simulink model "Copy_of_PROTOTIP_FULL2_plus_schema"  (R2022b)
settings: Solver=VariableStepAuto  StartTime=0.0  StopTime=5  FixedStep=1  RelTol=1e-3
model workspace (MAT data in the model file):
  K = Simulink.Parameter
  K.DataType = 'auto'
  K.Complexity = 'real'
  K.Dimensions = [0 0]
  K_v = Simulink.Parameter
  K_v.DataType = 'auto'
  K_v.Complexity = 'real'
  K_v.Dimensions = [0 0]
  Kp = Simulink.Parameter
  Kp.DataType = 'auto'
  Kp.Complexity = 'real'
  Kp.Dimensions = [0 0]
  Kv = Simulink.Parameter
  Kv.DataType = 'auto'
  Kv.Complexity = 'real'
  Kv.Dimensions = [0 0]
  Multiply1 = 1
  T2 = Simulink.Parameter
  T2.DataType = 'auto'
  T2.Complexity = 'real'
  T2.Dimensions = [0 0]
  W = Simulink.Parameter
  W.DataType = 'auto'
  W.Complexity = 'real'
  W.Dimensions = [0 0]
  q2dor = Simulink.Parameter
  q2dor.DataType = 'auto'
  q2dor.Complexity = 'real'
  q2dor.Dimensions = [0 0]
  q_1 = Simulink.Parameter
  q_1.Value = 1
  q_1.DataType = 'auto'
  q_1.Complexity = 'real'
  q_1.Dimensions = [1 1]
  q_1dor = Simulink.Parameter
  q_1dor.Value = 1
  q_1dor.DataType = 'auto'
  q_1dor.Complexity = 'real'
  q_1dor.Dimensions = [1 1]
  q_2dor = Simulink.Parameter
  q_2dor.Value = 1
  q_2dor.DataType = 'auto'
  q_2dor.Complexity = 'real'
  q_2dor.Dimensions = [1 1]
undefined symbols (not defined in the file or in its folder): X, Y, Z
libraries: sm_lib x17, nesl_utility x7
settings Model: Creator=Dell  LastModifiedBy=Dell
settings SimscapeCC: ExplicitSolverDiagnosticOptions=none

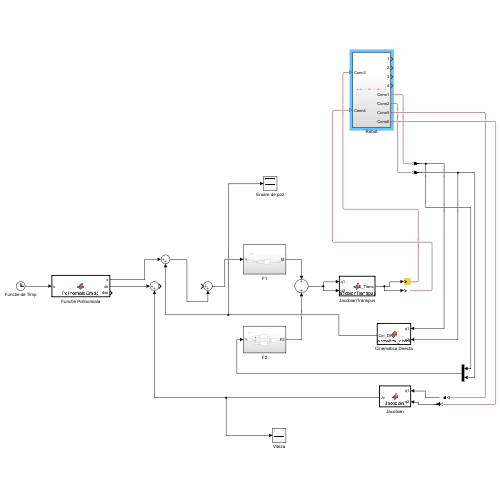
[thumbnail: Simulink's stored preview of the top-level diagram]
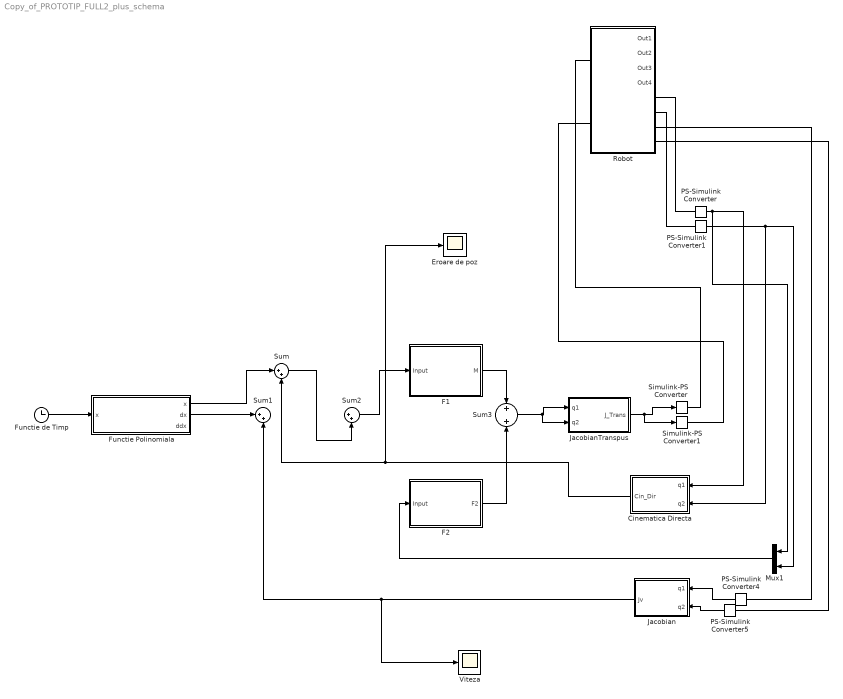
== system Copy_of_PROTOTIP_FULL2_plus_schema ==
  Cinematica Directa : MATLAB Function  TreatAsAtomicUnit=on
  Eroare de poz : Scope
  F1 : Subsystem
  F2 : Subsystem
  Functie Polinomiala : MATLAB Function  TreatAsAtomicUnit=on
  Functie de Timp : Clock
  Jacobian : MATLAB Function  TreatAsAtomicUnit=on
  JacobianTranspus : MATLAB Function  TreatAsAtomicUnit=on
  Mux1 : Mux  Inputs=2
  PS-Simulink Converter{,1,4..5} (4 alike) : nesl_utility/PS-Simulink Converter  PhysicalDomain=network_engine_domain  SubClassName=ps_output  LeftPortType=input  RightPortType=output  PseudoPeriodic=off  Frequencies=[]  VectorFormat=inherit  Unit=inherit  AffineConversion=off
  Robot : Subsystem
  Simulink-PS Converter : nesl_utility/Simulink-PS Converter  PhysicalDomain=network_engine_domain  SubClassName=ps_input  LeftPortType=input  RightPortType=output  PseudoPeriodic=off  Frequencies=[]  NoiseDistribution=none  NoiseParameters=[]  Unit=1  AffineConversion=on  FilteringAndDerivatives=provide  SimscapeFilterOrder=1  InputFilterTimeConstant=0.001  UdotUserProvided=0
  Simulink-PS Converter1 : nesl_utility/Simulink-PS Converter  PhysicalDomain=network_engine_domain  SubClassName=ps_input  LeftPortType=input  RightPortType=output  PseudoPeriodic=off  Frequencies=[]  NoiseDistribution=none  NoiseParameters=[]  Unit=1  AffineConversion=on  FilteringAndDerivatives=provide  SimscapeFilterOrder=1  InputFilterTimeConstant=0.001  UdotUserProvided=0
  Sum : Sum  Inputs=|++
  Sum1 : Sum  Inputs=|++
  Sum2 : Sum  Inputs=|++
  Sum3 : Sum  OutDataTypeStr=Inherit: Same as first input
  Viteza : Scope
  wires:
  Functie de Timp/1 -> Functie Polinomiala/1("x ")
  Functie Polinomiala/1(x) -> Sum/1
  F1/1(M) -> Sum3/1
  F2/1(F2) -> Sum3/2
  PS-Simulink Converter/1 -> Mux1/1, Cinematica Directa/1(q1)
  Cinematica Directa/1(Cin_Dir) -> Sum/2, Eroare de poz/1
  PS-Simulink Converter1/1 -> Mux1/2, Cinematica Directa/2(q2)
  Mux1/1 -> F2/1(Input)
  PS-Simulink Converter4/1 -> Jacobian/1(q1)
  PS-Simulink Converter5/1 -> Jacobian/2(q2)
  Functie Polinomiala/2(dx) -> Sum1/1
  Jacobian/1(Jv) -> Viteza/1, Sum1/2
  Sum2/1 -> F1/1(Input)
  JacobianTranspus/1(J_Trans) -> Simulink-PS Converter1/1, Simulink-PS Converter/1
  Sum/1 -> Sum2/2
  Sum3/1 -> JacobianTranspus/2(q2), JacobianTranspus/1(q1)
  connections:
  Simulink-PS Converter/RConn1 -- Robot/LConn1
  Simulink-PS Converter1/RConn1 -- Robot/LConn2
  PS-Simulink Converter/LConn1 -- Robot/RConn1
  Robot/RConn2 -- PS-Simulink Converter1/LConn1
  Robot/RConn3 -- PS-Simulink Converter4/LConn1
  Robot/RConn4 -- PS-Simulink Converter5/LConn1

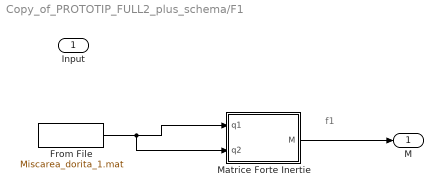
== system Copy_of_PROTOTIP_FULL2_plus_schema/F1 ==
  note: f1
  Input : Inport
  From File : FromFile  FileName=Miscarea_dorita_1.mat
  Matrice Forte Inertie : MATLAB Function  TreatAsAtomicUnit=on
  M : Outport
  wires:
  Matrice Forte Inertie/1(M) -> M/1
  From File/1 -> Matrice Forte Inertie/2(q2), Matrice Forte Inertie/1(q1)

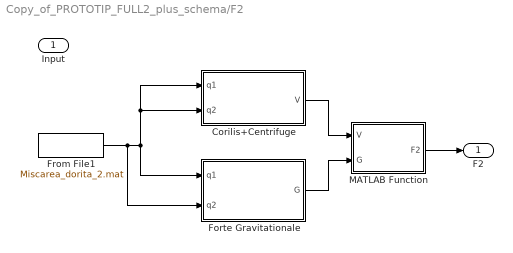
== system Copy_of_PROTOTIP_FULL2_plus_schema/F2 ==
  Input : Inport
  Corilis+Centrifuge : MATLAB Function  TreatAsAtomicUnit=on
  Forte Gravitationale : MATLAB Function  TreatAsAtomicUnit=on
  From File1 : FromFile  FileName=Miscarea_dorita_2.mat  SampleTime=0
  MATLAB Function : MATLAB Function  TreatAsAtomicUnit=on
  F2 : Outport
  wires:
  From File1/1 -> Forte Gravitationale/2(q2), Forte Gravitationale/1(q1), Corilis+Centrifuge/2(q2), Corilis+Centrifuge/1(q1)
  Corilis+Centrifuge/1(V) -> MATLAB Function/1(V)
  Forte Gravitationale/1(G) -> MATLAB Function/2(G)
  MATLAB Function/1(F2) -> F2/1

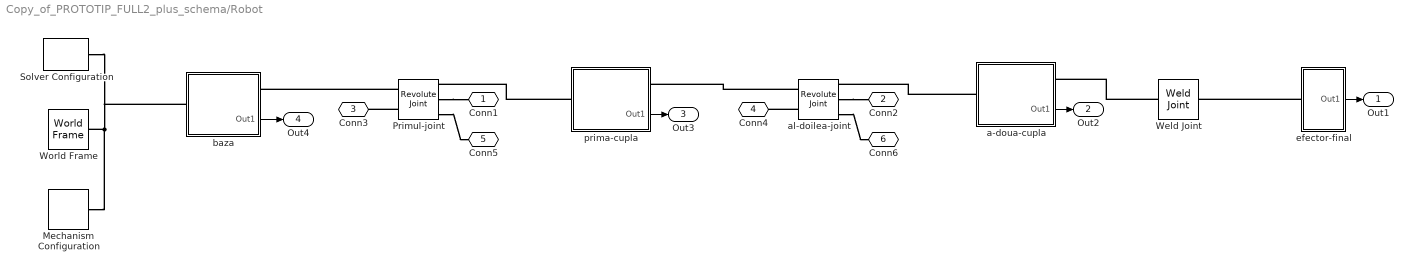
== system Copy_of_PROTOTIP_FULL2_plus_schema/Robot ==
  Mechanism Configuration : sm_lib/Utilities/Mechanism Configuration  UniformGravity=Constant  GravityVector=[0 0 -9.80665]  GravityUnits=m/s^2  LinearizationDelta=0.001  JointModeTransitionNonlinearIterations=2
  Primul-joint : sm_lib/Joints/Revolute Joint  JointMode=Normal  SenseConstraintForce=off  SenseConstraintForceX=off  SenseConstraintForceY=off  SenseConstraintForceZ=off  SenseConstraintTorque=off  SenseConstraintTorqueX=off  SenseConstraintTorqueY=off  SenseConstraintTorqueZ=off  SenseTotalForce=off  SenseTotalForceX=off  SenseTotalForceY=off  SenseTotalForceZ=off  SenseTotalTorque=off  SenseTotalTorqueX=off  SenseTotalTorqueY=off  SenseTotalTorqueZ=off  CompositeWrenchDir=FollowerOnBase  CompositeWrenchFrame=BaseFrame  EquilibriumPosition=0  EquilibriumPositionUnits=deg  SpringStiffness=0  SpringStiffnessUnits=N*m/deg  DampingCoefficient=0  DampingCoefficientUnits=N*m/(deg/s)  TorqueActuationMode=InputTorque  MotionActuationMode=ComputedMotion  SensePosition=on  SenseVelocity=on  SenseAcceleration=off  SenseTorqueForce=off  SenseLowerLimitTorqueForce=off  SenseUpperLimitTorqueForce=off  LowerLimitSpecify=off  LowerLimitBound=-90  LowerLimitBoundUnits=deg  LowerLimitStiffness=1e4  LowerLimitStiffnessUnits=N*m/deg  LowerLimitDamping=10  LowerLimitDampingUnits=N*m/(deg/s)  LowerLimitTransitionRegionWidth=0.1  LowerLimitTransitionRegionWidthUnits=deg  UpperLimitSpecify=off  UpperLimitBound=90  UpperLimitBoundUnits=deg  UpperLimitStiffness=1e4  UpperLimitStiffnessUnits=N*m/deg  UpperLimitDamping=10  UpperLimitDampingUnits=N*m/(deg/s)  UpperLimitTransitionRegionWidth=0.1  UpperLimitTransitionRegionWidthUnits=deg  PositionTargetSpecify=off  PositionTargetPriority=High  PositionTargetValue=0  PositionTargetValueUnits=deg  VelocityTargetSpecify=off  VelocityTargetPriority=High  VelocityTargetValue=0  VelocityTargetValueUnits=deg/s
  Solver Configuration : nesl_utility/Solver Configuration  PhysicalDomain=network_engine_domain  SubClassName=solver  LeftPortType=input  RightPortType=generic  Tones=[]  Harmonics=[]  SimulateNoise=off  Profile=off  UseLocalSampling=off  EnableSwitchedLinearOptims=on  FrequencyDomain=off  UseCCode=off  RelTol=0.001  AbsTol=0.001  MinStep=1e-09  ToWorkspace=off  RevertToSquareIcSolve=off  NumHomotopyIterations=100  PhasorMode=off  PhasorModeNumHarmonics=1  ConsistencySolver=NEWTON_XTOL_AFTER_FTOL  IndexReductionMethod=DerivativeReplacement  DoDC=off  ResidualTolerance=1e-09  ConsistencyTolSource=GLOBAL  ConsistencyAbsTol=0.001  ConsistencyRelTol=0.001  ConsistencyTolFactor=0.001  UseLocalSolver=off  LocalSolverChoice=NE_BACKWARD_EULER_ADVANCER  ResolveIndetEquations=on  FunctionEvalNumThread=1  LocalSolverSampleTime=0.001  DoFixedCost=off  MaxNonlinIter=3  MaxModeIter=2  ComputeImpulses=off  ImpulseIterations=2  LinearAlgebra=auto  LinearAlgebraNumThread=0  EquationFormulation=NE_TIME_EF  DelaysMemoryBudget=1024  AutomaticFiltering=on  FilteringTimeConstant=0.001  PartitionStorageMethod=AS_NEEDED  PartitionMemoryBudget=1024  PartitionMethod=ROBUST
  Weld Joint : sm_lib/Joints/Weld Joint  JointMode=Normal  SenseConstraintForce=off  SenseConstraintForceX=off  SenseConstraintForceY=off  SenseConstraintForceZ=off  SenseConstraintTorque=off  SenseConstraintTorqueX=off  SenseConstraintTorqueY=off  SenseConstraintTorqueZ=off  SenseTotalForce=off  SenseTotalForceX=off  SenseTotalForceY=off  SenseTotalForceZ=off  SenseTotalTorque=off  SenseTotalTorqueX=off  SenseTotalTorqueY=off  SenseTotalTorqueZ=off  CompositeWrenchDir=FollowerOnBase  CompositeWrenchFrame=BaseFrame
  World Frame : sm_lib/Frames and Transforms/World Frame
  a-doua-cupla : Subsystem
      settings: PortSchema="{\"entries\":[{\"content\":{\"sides\":[{\"content\":{\"connectorIds\":[\"LConn1\"]},\"type\":\"ConnectorPlacement.EquallySpacedRectSide\",\"uuid\":\"4c75c79d-8f02-4d38-9c7a-fb351d7c54a9\"},{\"content\":{\"connectorIds\":[\"RConn1\",\"Out1\"],\"side\":\"RIGHT\"},\"type\":\"ConnectorPlacement.EquallySpacedRectSide\",\"uuid\":\"34d13dc5-1ae9-4696-a3e2-997dd238e9eb\"},{\"content\":{\"connectorIds\":[],\"side\":\"TOP\"},\"type\":\"ConnectorPlacement.EquallySpacedRectSide\",\"uuid\":\"8a7d4810-dd50-497b-8594-43236fa50b5d\"}]},\"type\":\"ConnectorPlacement.EquallySpacedConnector\",\"uuid\":\"113eadfe-0302-4ebe-8106-46cacbe5f2bd\"}],\"packageUris\":[\"http://schema.mathworks.com/mf0/Connector/R2020b\"],\"version\":\"1.0\"}"
  al-doilea-joint : sm_lib/Joints/Revolute Joint  JointMode=Normal  SenseConstraintForce=off  SenseConstraintForceX=off  SenseConstraintForceY=off  SenseConstraintForceZ=off  SenseConstraintTorque=off  SenseConstraintTorqueX=off  SenseConstraintTorqueY=off  SenseConstraintTorqueZ=off  SenseTotalForce=off  SenseTotalForceX=off  SenseTotalForceY=off  SenseTotalForceZ=off  SenseTotalTorque=off  SenseTotalTorqueX=off  SenseTotalTorqueY=off  SenseTotalTorqueZ=off  CompositeWrenchDir=FollowerOnBase  CompositeWrenchFrame=BaseFrame  EquilibriumPosition=0  EquilibriumPositionUnits=deg  SpringStiffness=0  SpringStiffnessUnits=N*m/deg  DampingCoefficient=0  DampingCoefficientUnits=N*m/(deg/s)  TorqueActuationMode=InputTorque  MotionActuationMode=ComputedMotion  SensePosition=on  SenseVelocity=on  SenseAcceleration=off  SenseTorqueForce=off  SenseLowerLimitTorqueForce=off  SenseUpperLimitTorqueForce=off  LowerLimitSpecify=off  LowerLimitBound=-90  LowerLimitBoundUnits=deg  LowerLimitStiffness=1e4  LowerLimitStiffnessUnits=N*m/deg  LowerLimitDamping=10  LowerLimitDampingUnits=N*m/(deg/s)  LowerLimitTransitionRegionWidth=0.1  LowerLimitTransitionRegionWidthUnits=deg  UpperLimitSpecify=off  UpperLimitBound=90  UpperLimitBoundUnits=deg  UpperLimitStiffness=1e4  UpperLimitStiffnessUnits=N*m/deg  UpperLimitDamping=10  UpperLimitDampingUnits=N*m/(deg/s)  UpperLimitTransitionRegionWidth=0.1  UpperLimitTransitionRegionWidthUnits=deg  PositionTargetSpecify=off  PositionTargetPriority=High  PositionTargetValue=0  PositionTargetValueUnits=deg  VelocityTargetSpecify=off  VelocityTargetPriority=High  VelocityTargetValue=0  VelocityTargetValueUnits=deg/s
  baza : Subsystem
      settings: PortSchema="{\"entries\":[{\"content\":{\"sides\":[{\"content\":{\"connectorIds\":[\"LConn1\"]},\"type\":\"ConnectorPlacement.EquallySpacedRectSide\",\"uuid\":\"4c75c79d-8f02-4d38-9c7a-fb351d7c54a9\"},{\"content\":{\"connectorIds\":[\"RConn1\",\"Out1\"],\"side\":\"RIGHT\"},\"type\":\"ConnectorPlacement.EquallySpacedRectSide\",\"uuid\":\"34d13dc5-1ae9-4696-a3e2-997dd238e9eb\"},{\"content\":{\"connectorIds\":[],\"side\":\"TOP\"},\"type\":\"ConnectorPlacement.EquallySpacedRectSide\",\"uuid\":\"8a7d4810-dd50-497b-8594-43236fa50b5d\"}]},\"type\":\"ConnectorPlacement.EquallySpacedConnector\",\"uuid\":\"113eadfe-0302-4ebe-8106-46cacbe5f2bd\"}],\"packageUris\":[\"http://schema.mathworks.com/mf0/Connector/R2020b\"],\"version\":\"1.0\"}"
  efector-final : Subsystem
  prima-cupla : Subsystem
      settings: PortSchema="{\"entries\":[{\"content\":{\"sides\":[{\"content\":{\"connectorIds\":[\"LConn1\"]},\"type\":\"ConnectorPlacement.EquallySpacedRectSide\",\"uuid\":\"4c75c79d-8f02-4d38-9c7a-fb351d7c54a9\"},{\"content\":{\"connectorIds\":[\"RConn1\",\"Out1\"],\"side\":\"RIGHT\"},\"type\":\"ConnectorPlacement.EquallySpacedRectSide\",\"uuid\":\"34d13dc5-1ae9-4696-a3e2-997dd238e9eb\"},{\"content\":{\"connectorIds\":[],\"side\":\"TOP\"},\"type\":\"ConnectorPlacement.EquallySpacedRectSide\",\"uuid\":\"8a7d4810-dd50-497b-8594-43236fa50b5d\"}]},\"type\":\"ConnectorPlacement.EquallySpacedConnector\",\"uuid\":\"113eadfe-0302-4ebe-8106-46cacbe5f2bd\"}],\"packageUris\":[\"http://schema.mathworks.com/mf0/Connector/R2020b\"],\"version\":\"1.0\"}"
  Conn1 : PMIOPort  Side=Right
  Conn2 : PMIOPort  Port=2  Side=Right
  Conn3 : PMIOPort  Port=3  Side=Left
  Conn4 : PMIOPort  Port=4  Side=Left
  Conn5 : PMIOPort  Port=5  Side=Right
  Conn6 : PMIOPort  Port=6  Side=Right
  Out1 : Outport
  Out2 : Outport  Port=2
  Out3 : Outport  Port=3
  Out4 : Outport  Port=4
  wires:
  baza/1(Out1) -> Out4/1
  prima-cupla/1(Out1) -> Out3/1
  a-doua-cupla/1(Out1) -> Out2/1
  efector-final/1(Out1) -> Out1/1
  connections:
  Mechanism Configuration/RConn1 -- Solver Configuration/RConn1 -- baza/LConn1 -- World Frame/RConn1
  prima-cupla/LConn1 -- Primul-joint/RConn1
  a-doua-cupla/LConn1 -- al-doilea-joint/RConn1
  efector-final/LConn1 -- Weld Joint/RConn1
  Weld Joint/LConn1 -- a-doua-cupla/RConn1
  al-doilea-joint/LConn1 -- prima-cupla/RConn1
  Primul-joint/LConn1 -- baza/RConn1
  al-doilea-joint/RConn2 -- Conn2/RConn1
  al-doilea-joint/RConn3 -- Conn6/RConn1
  Primul-joint/LConn2 -- Conn3/RConn1
  Primul-joint/RConn3 -- Conn5/RConn1
  Primul-joint/RConn2 -- Conn1/RConn1
  al-doilea-joint/LConn2 -- Conn4/RConn1

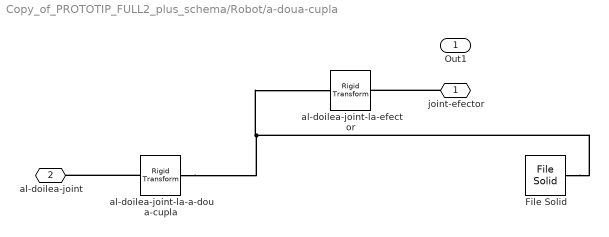
== system Copy_of_PROTOTIP_FULL2_plus_schema/Robot/a-doua-cupla ==
  File Solid : sm_lib/Body Elements/File Solid  ExtGeomFileName=C:\Users\Dell\Desktop\Anul III\Semestrul II Anul III\SCR\Cursuri\A_Doua_Cupla.CATPart  UnitType=FromFile  ExtGeomFileUnits=m  StepReaderType=HEX  ExportConvexHullGeometry=off  InertiaType=CalculateFromGeometry  Mass=1  MassUnits=kg  CenterOfMass=[0 0 0]  CenterOfMassUnits=m  MomentsOfInertia=[1 1 1]  MomentsOfInertiaUnits=kg*m^2  ProductsOfInertia=[0 0 0]  ProductsOfInertiaUnits=kg*m^2  BasedOnType=DensityFromFile  Density=1000  DensityUnits=kg/m^3  DoExposeReferenceFrame=on  SerializedFrames=<Frames/>  GraphicType=FromGeometry  MarkerShape=Sphere  MarkerSize=10  GraphicVisPropType=SimpleVisualProperties  GraphicDiffuseColor=[0.5 0.5 0.5]  GraphicSpecularColor=[0.5 0.5 0.5 1.0]  GraphicAmbientColor=[0.15 0.15 0.15 1.0]  GraphicEmissiveColor=[0.0 0.0 0.0 1.0]  GraphicShininess=75  GraphicOpacity=1.0
  al-doilea-joint-la-a-doua-cupla : sm_lib/Frames and Transforms/Rigid Transform  TranslationMethod=Cartesian  TranslationStandardOffset=0  TranslationLengthUnit=mm  TranslationStandardAxis=+Z  TranslationCartesianOffset=[50 -52 -5]  TranslationROffset=0  TranslationROffsetUnits=m  TranslationZOffset=0  TranslationZOffsetUnits=m  TranslationThetaOffset=0  TranslationThetaOffsetUnits=deg  RotationMethod=None  RotationAngleUnits=deg  RotationStandardAxis=+Z  RotationAngle=0.0  RotationArbitraryAxis=[0 0 1]  FollAlignAxisA=+X  BaseAlignAxisA=+Y  FollAlignAxisB=+Y  BaseAlignAxisB=+Z  RotationSequenceAxes=FollowerAxes  RotationSequence=XYX  RotationSequenceAngles=[0 0 0]  RotationSequenceAnglesUnits=deg  RotationMatrix=[1 0 0; 0 1 0; 0 0 1]  Quaternion=[1 0 0 0]
  al-doilea-joint-la-efector : sm_lib/Frames and Transforms/Rigid Transform  TranslationMethod=Cartesian  TranslationStandardOffset=0  TranslationLengthUnit=m  TranslationStandardAxis=+Z  TranslationCartesianOffset=[0.075 0 0]  TranslationROffset=0  TranslationROffsetUnits=m  TranslationZOffset=0  TranslationZOffsetUnits=m  TranslationThetaOffset=0  TranslationThetaOffsetUnits=deg  RotationMethod=None  RotationAngleUnits=deg  RotationStandardAxis=+Z  RotationAngle=0.0  RotationArbitraryAxis=[0 0 1]  FollAlignAxisA=+X  BaseAlignAxisA=+Y  FollAlignAxisB=+Y  BaseAlignAxisB=+Z  RotationSequenceAxes=FollowerAxes  RotationSequence=XYX  RotationSequenceAngles=[0 0 0]  RotationSequenceAnglesUnits=deg  RotationMatrix=[1 0 0; 0 1 0; 0 0 1]  Quaternion=[1 0 0 0]
  joint-efector : PMIOPort  Side=Right
  al-doilea-joint : PMIOPort  Port=2  Side=Left
  Out1 : Outport
  connections:
  File Solid/RConn1 -- al-doilea-joint-la-a-doua-cupla/RConn1 -- al-doilea-joint-la-efector/LConn1
  al-doilea-joint-la-a-doua-cupla/LConn1 -- al-doilea-joint/RConn1
  joint-efector/RConn1 -- al-doilea-joint-la-efector/RConn1

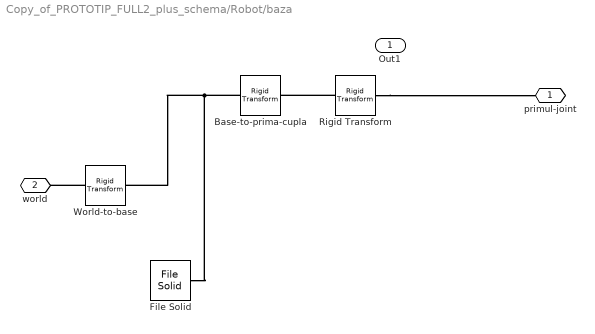
== system Copy_of_PROTOTIP_FULL2_plus_schema/Robot/baza ==
  Base-to-prima-cupla : sm_lib/Frames and Transforms/Rigid Transform  TranslationMethod=StandardAxis  TranslationStandardOffset=100  TranslationLengthUnit=mm  TranslationStandardAxis=-X  TranslationCartesianOffset=[0 0 0]  TranslationROffset=0  TranslationROffsetUnits=m  TranslationZOffset=0  TranslationZOffsetUnits=m  TranslationThetaOffset=0  TranslationThetaOffsetUnits=deg  RotationMethod=None  RotationAngleUnits=deg  RotationStandardAxis=+X  RotationAngle=180  RotationArbitraryAxis=[0 0 1]  FollAlignAxisA=+X  BaseAlignAxisA=+Y  FollAlignAxisB=+Y  BaseAlignAxisB=+Z  RotationSequenceAxes=FollowerAxes  RotationSequence=XYX  RotationSequenceAngles=[0 0 0]  RotationSequenceAnglesUnits=deg  RotationMatrix=[1 0 0; 0 1 0; 0 0 1]  Quaternion=[1 0 0 0]
  File Solid : sm_lib/Body Elements/File Solid  ExtGeomFileName=C:\Users\Dell\Desktop\Anul III\Semestrul II Anul III\SCR\Cursuri\Base.CATPart  UnitType=FromFile  ExtGeomFileUnits=m  StepReaderType=HEX  ExportConvexHullGeometry=off  InertiaType=CalculateFromGeometry  Mass=1  MassUnits=kg  CenterOfMass=[0 0 0]  CenterOfMassUnits=m  MomentsOfInertia=[1 1 1]  MomentsOfInertiaUnits=kg*m^2  ProductsOfInertia=[0 0 0]  ProductsOfInertiaUnits=kg*m^2  BasedOnType=DensityFromFile  Density=1000  DensityUnits=kg/m^3  DoExposeReferenceFrame=on  SerializedFrames=<Frames/>  GraphicType=FromGeometry  MarkerShape=Sphere  MarkerSize=10  GraphicVisPropType=SimpleVisualProperties  GraphicDiffuseColor=[0.5 0.5 0.5]  GraphicSpecularColor=[0.5 0.5 0.5 1.0]  GraphicAmbientColor=[0.15 0.15 0.15 1.0]  GraphicEmissiveColor=[0.0 0.0 0.0 1.0]  GraphicShininess=75  GraphicOpacity=1.0
  Rigid Transform : sm_lib/Frames and Transforms/Rigid Transform  TranslationMethod=StandardAxis  TranslationStandardOffset=-12  TranslationLengthUnit=mm  TranslationStandardAxis=+Z  TranslationCartesianOffset=[0 0 0]  TranslationROffset=0  TranslationROffsetUnits=m  TranslationZOffset=0  TranslationZOffsetUnits=m  TranslationThetaOffset=0  TranslationThetaOffsetUnits=deg  RotationMethod=None  RotationAngleUnits=deg  RotationStandardAxis=+Z  RotationAngle=0.0  RotationArbitraryAxis=[0 0 1]  FollAlignAxisA=+X  BaseAlignAxisA=+Y  FollAlignAxisB=+Y  BaseAlignAxisB=+Z  RotationSequenceAxes=FollowerAxes  RotationSequence=XYX  RotationSequenceAngles=[0 0 0]  RotationSequenceAnglesUnits=deg  RotationMatrix=[1 0 0; 0 1 0; 0 0 1]  Quaternion=[1 0 0 0]
  World-to-base : sm_lib/Frames and Transforms/Rigid Transform  TranslationMethod=StandardAxis  TranslationStandardOffset=100  TranslationLengthUnit=mm  TranslationStandardAxis=-X  TranslationCartesianOffset=[0 0 0]  TranslationROffset=0  TranslationROffsetUnits=m  TranslationZOffset=0  TranslationZOffsetUnits=m  TranslationThetaOffset=0  TranslationThetaOffsetUnits=deg  RotationMethod=StandardAxis  RotationAngleUnits=deg  RotationStandardAxis=+X  RotationAngle=180  RotationArbitraryAxis=[0 0 1]  FollAlignAxisA=+X  BaseAlignAxisA=+Y  FollAlignAxisB=+Y  BaseAlignAxisB=+Z  RotationSequenceAxes=FollowerAxes  RotationSequence=XYX  RotationSequenceAngles=[0 0 0]  RotationSequenceAnglesUnits=deg  RotationMatrix=[1 0 0; 0 1 0; 0 0 1]  Quaternion=[1 0 0 0]
  primul-joint : PMIOPort  Side=Right
  world : PMIOPort  Port=2  Side=Left
  Out1 : Outport
  connections:
  Base-to-prima-cupla/LConn1 -- File Solid/RConn1 -- World-to-base/RConn1
  World-to-base/LConn1 -- world/RConn1
  Rigid Transform/LConn1 -- Base-to-prima-cupla/RConn1
  Rigid Transform/RConn1 -- primul-joint/RConn1

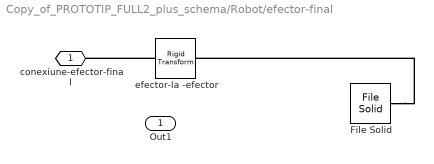
== system Copy_of_PROTOTIP_FULL2_plus_schema/Robot/efector-final ==
  File Solid : sm_lib/Body Elements/File Solid  ExtGeomFileName=C:\Users\Dell\Desktop\Anul III\Semestrul II Anul III\SCR\Cursuri\End-EfectorCATPart.CATPart  UnitType=FromFile  ExtGeomFileUnits=m  StepReaderType=HEX  ExportConvexHullGeometry=off  InertiaType=CalculateFromGeometry  Mass=1  MassUnits=kg  CenterOfMass=[0 0 0]  CenterOfMassUnits=m  MomentsOfInertia=[1 1 1]  MomentsOfInertiaUnits=kg*m^2  ProductsOfInertia=[0 0 0]  ProductsOfInertiaUnits=kg*m^2  BasedOnType=DensityFromFile  Density=1000  DensityUnits=kg/m^3  DoExposeReferenceFrame=on  SerializedFrames=<Frames/>  GraphicType=FromGeometry  MarkerShape=Sphere  MarkerSize=10  GraphicVisPropType=SimpleVisualProperties  GraphicDiffuseColor=[0.5 0.5 0.5]  GraphicSpecularColor=[0.5 0.5 0.5 1.0]  GraphicAmbientColor=[0.15 0.15 0.15 1.0]  GraphicEmissiveColor=[0.0 0.0 0.0 1.0]  GraphicShininess=75  GraphicOpacity=1.0
  efector-la -efector : sm_lib/Frames and Transforms/Rigid Transform  TranslationMethod=Cartesian  TranslationStandardOffset=0  TranslationLengthUnit=mm  TranslationStandardAxis=+Z  TranslationCartesianOffset=[5 0 30]  TranslationROffset=0  TranslationROffsetUnits=m  TranslationZOffset=0  TranslationZOffsetUnits=m  TranslationThetaOffset=0  TranslationThetaOffsetUnits=deg  RotationMethod=StandardAxis  RotationAngleUnits=deg  RotationStandardAxis=+Y  RotationAngle=180  RotationArbitraryAxis=[0 0 1]  FollAlignAxisA=+X  BaseAlignAxisA=+Y  FollAlignAxisB=+Y  BaseAlignAxisB=+Z  RotationSequenceAxes=FollowerAxes  RotationSequence=XYX  RotationSequenceAngles=[0 0 0]  RotationSequenceAnglesUnits=deg  RotationMatrix=[1 0 0; 0 1 0; 0 0 1]  Quaternion=[1 0 0 0]
  conexiune-efector-final : PMIOPort  Side=Left
  Out1 : Outport
  connections:
  File Solid/RConn1 -- efector-la -efector/RConn1
  efector-la -efector/LConn1 -- conexiune-efector-final/RConn1

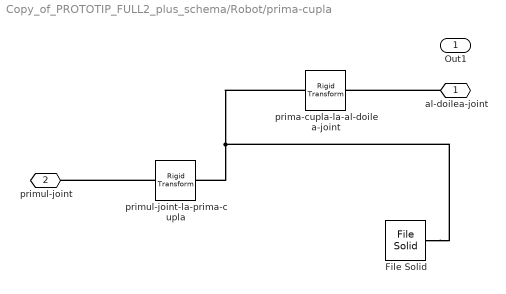
== system Copy_of_PROTOTIP_FULL2_plus_schema/Robot/prima-cupla ==
  File Solid : sm_lib/Body Elements/File Solid  ExtGeomFileName=C:\Users\Dell\Desktop\Anul III\Semestrul II Anul III\SCR\Cursuri\Prima_Cupla.CATPart  UnitType=FromFile  ExtGeomFileUnits=m  StepReaderType=HEX  ExportConvexHullGeometry=off  InertiaType=CalculateFromGeometry  Mass=1  MassUnits=kg  CenterOfMass=[0 0 0]  CenterOfMassUnits=m  MomentsOfInertia=[1 1 1]  MomentsOfInertiaUnits=kg*m^2  ProductsOfInertia=[0 0 0]  ProductsOfInertiaUnits=kg*m^2  BasedOnType=DensityFromFile  Density=1000  DensityUnits=kg/m^3  DoExposeReferenceFrame=on  SerializedFrames=<Frames/>  GraphicType=FromGeometry  MarkerShape=Sphere  MarkerSize=10  GraphicVisPropType=SimpleVisualProperties  GraphicDiffuseColor=[0.5 0.5 0.5]  GraphicSpecularColor=[0.5 0.5 0.5 1.0]  GraphicAmbientColor=[0.15 0.15 0.15 1.0]  GraphicEmissiveColor=[0.0 0.0 0.0 1.0]  GraphicShininess=75  GraphicOpacity=1.0
  prima-cupla-la-al-doilea-joint : sm_lib/Frames and Transforms/Rigid Transform  TranslationMethod=Cartesian  TranslationStandardOffset=-30  TranslationLengthUnit=mm  TranslationStandardAxis=+X  TranslationCartesianOffset=[9 0 0]  TranslationROffset=0  TranslationROffsetUnits=m  TranslationZOffset=0  TranslationZOffsetUnits=m  TranslationThetaOffset=0  TranslationThetaOffsetUnits=deg  RotationMethod=StandardAxis  RotationAngleUnits=deg  RotationStandardAxis=+Z  RotationAngle=45  RotationArbitraryAxis=[0 0 1]  FollAlignAxisA=+X  BaseAlignAxisA=+Y  FollAlignAxisB=+Y  BaseAlignAxisB=+Z  RotationSequenceAxes=FollowerAxes  RotationSequence=XYX  RotationSequenceAngles=[0 0 0]  RotationSequenceAnglesUnits=deg  RotationMatrix=[1 0 0; 0 1 0; 0 0 1]  Quaternion=[1 0 0 0]
  primul-joint-la-prima-cupla : sm_lib/Frames and Transforms/Rigid Transform  TranslationMethod=Cartesian  TranslationStandardOffset=0  TranslationLengthUnit=m  TranslationStandardAxis=+Z  TranslationCartesianOffset=[0.1 0 0]  TranslationROffset=0  TranslationROffsetUnits=m  TranslationZOffset=0  TranslationZOffsetUnits=m  TranslationThetaOffset=0  TranslationThetaOffsetUnits=deg  RotationMethod=None  RotationAngleUnits=deg  RotationStandardAxis=+Z  RotationAngle=0.0  RotationArbitraryAxis=[0 0 1]  FollAlignAxisA=+X  BaseAlignAxisA=+Y  FollAlignAxisB=+Y  BaseAlignAxisB=+Z  RotationSequenceAxes=FollowerAxes  RotationSequence=XYX  RotationSequenceAngles=[0 0 0]  RotationSequenceAnglesUnits=deg  RotationMatrix=[1 0 0; 0 1 0; 0 0 1]  Quaternion=[1 0 0 0]
  al-doilea-joint : PMIOPort  Side=Right
  primul-joint : PMIOPort  Port=2  Side=Left
  Out1 : Outport
  connections:
  prima-cupla-la-al-doilea-joint/LConn1 -- primul-joint-la-prima-cupla/RConn1 -- File Solid/RConn1
  primul-joint-la-prima-cupla/LConn1 -- primul-joint/RConn1
  al-doilea-joint/RConn1 -- prima-cupla-la-al-doilea-joint/RConn1

== matlab function Copy_of_PROTOTIP_FULL2_plus_schema/Jacobian ==
  data: q1 input; Jv output; q2 input
function  Jv= Jacobian(q1,q2)

l1=1;
l2=2;

Jv=[l1*sin(q1)-l2*sin(q1+q2) , -l2*sin(q1+q2);
    l1*cos(q1)-l2*cos(q1+q2) , l2*cos(q1+q2)];

== matlab function Copy_of_PROTOTIP_FULL2_plus_schema/F2/MATLAB Function ==
  data: V input; F2 output; G input
function F2 = fcn(V,G)

F2=V+G;

== matlab function Copy_of_PROTOTIP_FULL2_plus_schema/F1/Matrice Forte Inertie ==
  data: q1 input; M output; q2 input
function M = MatriceInertie(q1,q2)

l1=1;
l2=1;
m1=0.5;
m2=0.5;
I_zz_1=0.3;
I_zz_2=0.2;

M=[m1*l1+m2*l1+m2*l2+2*m2*l1*l2*sin(q1)+I_zz_1 , m2*(l2^2)+I_zz_2;
    m2*(l2^2)+m2*l1*l2*cos(q2)+I_zz_2 , m2*(l2^2)+I_zz_2];

== matlab function Copy_of_PROTOTIP_FULL2_plus_schema/F2/Corilis+Centrifuge ==
  data: V output; q1 input; q2 input
function V = CoriolisCentrifuge(q1,q2)

l1=1;
l2=1;
m2=0.5;
%matrice centrifuge

C=[0 , -m2*l1*l2*sin(q1);
    -m2*l1*l2*sin(q2), 0];

%matrice coriolis

B =[-2*m2*l1*l2*sin(q2),0;
    0,0];
V = C+B;

== matlab function Copy_of_PROTOTIP_FULL2_plus_schema/F2/Forte Gravitationale ==
  data: q1 input; G output; q2 input
function G = ForteGravitationale(q1,q2)

m1=0.5;
m2=0.5;
g=9.81;
l1=1;
l2=1;

G=[m1*g+m2*g-l1*sin(q1) , m1*g+m2*g-l1*sin(q1)+l2*cos(q2);
    0,0];

== matlab function Copy_of_PROTOTIP_FULL2_plus_schema/JacobianTranspus ==
  data: q1 input; J_Trans output; q2 input
function J_Trans = JacobianTranspus(q1,q2)

l1=1;
l2=1;

J_Trans=[l1*cos(q1)-l2*cos(q1+q2) , l1*sin(q1)-l2*sin(q1+q2) ;
    -l2*cos(q1+q2) ,l2*sin(q1+q2)];

== matlab function Copy_of_PROTOTIP_FULL2_plus_schema/Cinematica Directa ==
  data: q1 input; Cin_Dir output; q2 input
function Cin_Dir = Cinematica_directa(q1,q2)

l_1=1;
l_2=2;
Cin_Dir=[l_1*cos(q1)+l_2*cos(q1+q2);
    l_1*sin(q1)+l_2*sin(q1+q2);];

== matlab function Copy_of_PROTOTIP_FULL2_plus_schema/Functie Polinomiala ==
  data: x input; x output; dx output; ddx output
function [x, dx, ddx] = PolinomialaGrad3(x)
    

    

    
    a = 1;
    b = 2;
    c = 3;
    d = 4;

    
    x = a * x^3 + b * x^2 + c * x + d;
    dx = 3 * a * x^2 + 2 * b * x + c;
    ddx = 6 * a * x + 2 * b;

end
